simulink model "simulink_model"  (R2021b)
settings: Solver=VariableStepAuto  StartTime=0.0  StopTime=3  RelTol=1e-3
values from neighbouring files (symbols this model uses):
  alpha_A0 = pi/6    (= 0.523598775598)    [constants.m]
  alpha_D0 = pi    (= 3.14159265359)    [constants.m]
  alpha_T0 = 7*pi/6    (= 3.66519142919)    [constants.m]
  R_DT0 = sqrt((xD0 - xT0)^2 + (yD0 - yT0)^2)    [constants.m]
  R_TA0 = sqrt((xA0 - xT0)^2 + (yA0 - yT0)^2)    [constants.m]
  theta_DT0 = atan2(yD0 - yT0,xD0 - xT0)    [constants.m]
  theta_TA0 = atan2(yA0 - yT0,xA0 - xT0)    [constants.m]
  xT0 = -5    [constants.m]
  yT0 = 20    [constants.m]
settings Model: SimulationMode=accelerator  Creator=dhruv  LastModifiedBy=dhruv

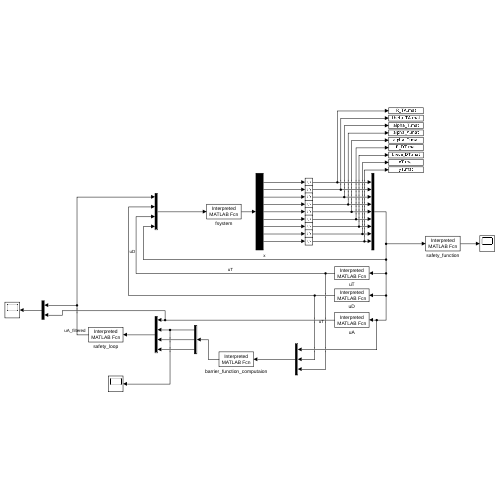
[thumbnail: Simulink's stored preview of the top-level diagram]
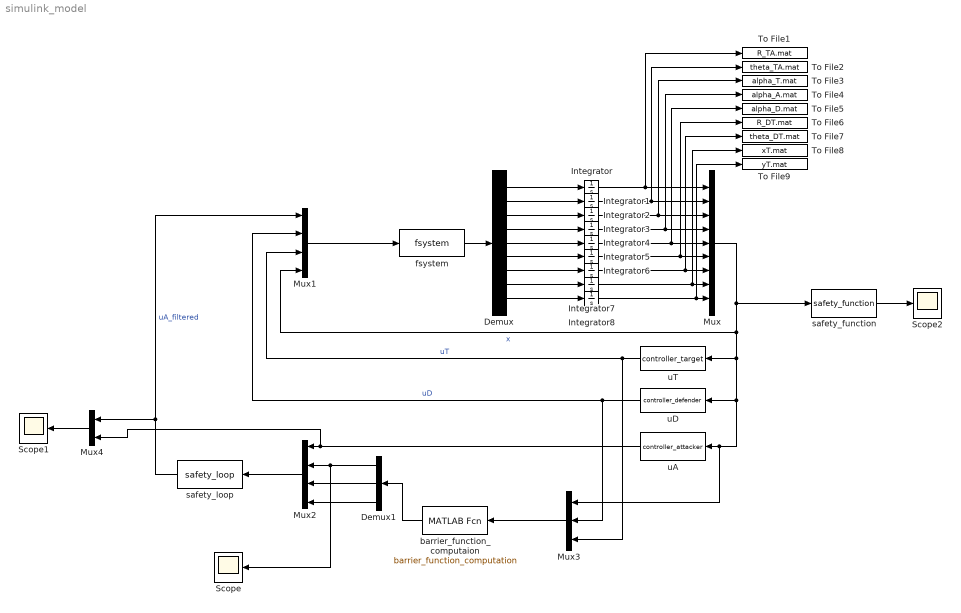
== system simulink_model ==
  Demux : Demux  Outputs=9
  Demux1 : Demux  Outputs=3
  Integrator : Integrator  InitialCondition=R_TA0
  Integrator1 : Integrator  InitialCondition=theta_TA0
  Integrator2 : Integrator  InitialCondition=alpha_T0
  Integrator3 : Integrator  InitialCondition=alpha_A0
  Integrator4 : Integrator  InitialCondition=alpha_D0
  Integrator5 : Integrator  InitialCondition=R_DT0
  Integrator6 : Integrator  InitialCondition=theta_DT0
  Integrator7 : Integrator  InitialCondition=xT0
  Integrator8 : Integrator  InitialCondition=yT0
  Mux : Mux  Inputs=9
  Mux1 : Mux
  Mux2 : Mux
  Mux3 : Mux  Inputs=3
  Mux4 : Mux  Inputs=2
  Scope : Scope
  Scope1 : Scope
  Scope2 : Scope
  To File1 : ToFile  Filename=R_TA.mat  MatrixName=R_TA  SaveFormat=Timeseries
  To File2 : ToFile  Filename=theta_TA.mat  MatrixName=theta_TA  SaveFormat=Timeseries
  To File3 : ToFile  Filename=alpha_T.mat  MatrixName=alpha_T  SaveFormat=Timeseries
  To File4 : ToFile  Filename=alpha_A.mat  MatrixName=alpha_A  SaveFormat=Timeseries
  To File5 : ToFile  Filename=alpha_D.mat  MatrixName=alpha_D  SaveFormat=Timeseries
  To File6 : ToFile  Filename=R_DT.mat  MatrixName=R_DT  SaveFormat=Timeseries
  To File7 : ToFile  Filename=theta_DT.mat  MatrixName=theta_DT  SaveFormat=Timeseries
  To File8 : ToFile  Filename=xT.mat  MatrixName=xT  SaveFormat=Timeseries
  To File9 : ToFile  Filename=yT.mat  MatrixName=yT  SaveFormat=Timeseries
  barrier_function_computaion : MATLABFcn  MATLABFcn=barrier_function_computation  OutputDimensions=3
  fsystem : MATLABFcn  MATLABFcn=fsystem  OutputDimensions=9
  safety_function : MATLABFcn  MATLABFcn=safety_function  OutputDimensions=2
  safety_loop : MATLABFcn  MATLABFcn=safety_loop  OutputDimensions=1
  uA : MATLABFcn  MATLABFcn=controller_attacker  OutputDimensions=1
  uD : MATLABFcn  MATLABFcn=controller_defender  OutputDimensions=1
  uT : MATLABFcn  MATLABFcn=controller_target  OutputDimensions=1
  wires:
  fsystem/1 -> Demux/1
  Demux/1 -> Integrator/1
  Demux/2 -> Integrator1/1
  Demux/3 -> Integrator2/1
  Demux/4 -> Integrator3/1
  Demux/5 -> Integrator4/1
  Demux/6 -> Integrator5/1
  Demux/7 -> Integrator6/1
  Demux/8 -> Integrator7/1
  Demux/9 -> Integrator8/1
  Integrator/1 -> To File1/1, Mux/1
  Integrator1/1 -> To File2/1, Mux/2
  Integrator2/1 -> To File3/1, Mux/3
  Integrator3/1 -> To File4/1, Mux/4
  Integrator4/1 -> To File5/1, Mux/5
  Integrator5/1 -> To File6/1, Mux/6
  Integrator6/1 -> To File7/1, Mux/7
  Integrator7/1 -> To File8/1, Mux/8
  Integrator8/1 -> To File9/1, Mux/9
  Mux1/1 -> fsystem/1
  Mux/1 -> Mux3/1, uA/1, uD/1, uT/1, Mux1/4, safety_function/1  "x"
  safety_loop/1 -> Mux1/1, Mux4/1  "uA_filtered"
  uD/1 -> Mux3/2, Mux1/2  "uD"
  uT/1 -> Mux1/3, Mux3/3  "uT"
  Mux2/1 -> safety_loop/1
  barrier_function_computaion/1 -> Demux1/1
  Demux1/3 -> Mux2/4
  Demux1/2 -> Mux2/3
  Demux1/1 -> Scope/1, Mux2/2
  uA/1 -> Mux4/2, Mux2/1
  Mux3/1 -> barrier_function_computaion/1
  Mux4/1 -> Scope1/1
  safety_function/1 -> Scope2/1
